simulink model "Copy_of_Q7Speed_Controller"  (R2013a)
settings: Solver=ode45  StartTime=0.0  StopTime=0.5  MaxStep=1e-4  RelTol=1e-3
values from neighbouring files (symbols this model uses):
  Km = (P/2)*(Kt/Bt)    (= 37.1743988584)    [Q1.m]    (also in Q4.m; Q5.m; Q6.m; Q8.m)
  La = Ls-(Lm*Lm/Lr)    (= 0.00366889047449)    [Q1.m]    (also in Q4.m; Q5.m; Q6.m; Q8.m)
  Ls = 0.0553    [Q1.m]    (also in Q4.m; Q5.m; Q6.m; Q8.m)
  Ra = Rs+Rr*(Ls/Lr)    (= 0.457519086693)    [Q1.m]    (also in Q4.m; Q5.m; Q6.m; Q8.m)
  Tm = J/Bt    (= 0.33)    [Q1.m]    (also in Q4.m; Q5.m; Q6.m; Q8.m)
undefined symbols (not defined in the file or in its folder): ids
settings Model: Creator=Sony  LastModifiedBy=Sony

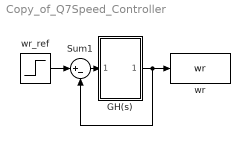
== system Copy_of_Q7Speed_Controller ==
  GH(s) : Subsystem
  Sum1 : Sum  Inputs=|+-
  wr : ToWorkspace  VariableName=wr  SampleTime=-1  SaveFormat=Timeseries
  wr_ref : Step  Time=0  After=1*0.05  SampleTime=0
  wires:
  wr_ref/1 -> Sum1/1
  Sum1/1 -> GH(s)/1(In1)
  GH(s)/1(Out1) -> Sum1/2, wr/1

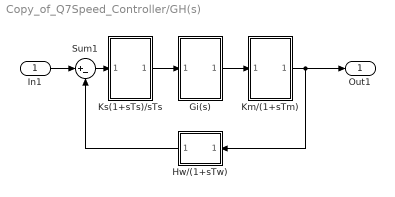
== system Copy_of_Q7Speed_Controller/GH(s) ==
  In1 : Inport
  Gi(s) : Subsystem
  Hw/(1+sTw) : Subsystem
  Km/(1+sTm) : Subsystem
  Ks(1+sTs)/sTs : Subsystem
  Sum1 : Sum  Inputs=|+-
  Out1 : Outport
  wires:
  In1/1 -> Sum1/1
  Km/(1+sTm)/1(Out1) -> Out1/1, Hw/(1+sTw)/1(In1)
  Ks(1+sTs)/sTs/1(Out1) -> Gi(s)/1(In1)
  Gi(s)/1(Out1) -> Km/(1+sTm)/1(In1)
  Hw/(1+sTw)/1(Out1) -> Sum1/2
  Sum1/1 -> Ks(1+sTs)/sTs/1(In1)

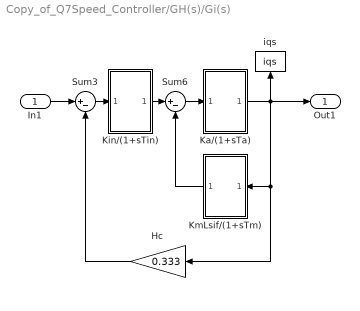
== system Copy_of_Q7Speed_Controller/GH(s)/Gi(s) ==
  In1 : Inport
  Hc : Gain  Gain=0.333
  Ka/(1+sTa) : Subsystem
  Kin/(1+sTin) : Subsystem
  KmLsif/(1+sTm) : Subsystem
  Sum3 : Sum  Inputs=|+-
  Sum6 : Sum  Inputs=|+-
  iqs : ToWorkspace  VariableName=iqs  SampleTime=-1  SaveFormat=Timeseries
  Out1 : Outport
  wires:
  Hc/1 -> Sum3/2
  In1/1 -> Sum3/1
  Sum6/1 -> Ka/(1+sTa)/1(In1)
  KmLsif/(1+sTm)/1(Out1) -> Sum6/2
  Ka/(1+sTa)/1(Out1) -> Out1/1, KmLsif/(1+sTm)/1(In1), Hc/1, iqs/1
  Sum3/1 -> Kin/(1+sTin)/1(In1)
  Kin/(1+sTin)/1(Out1) -> Sum6/1

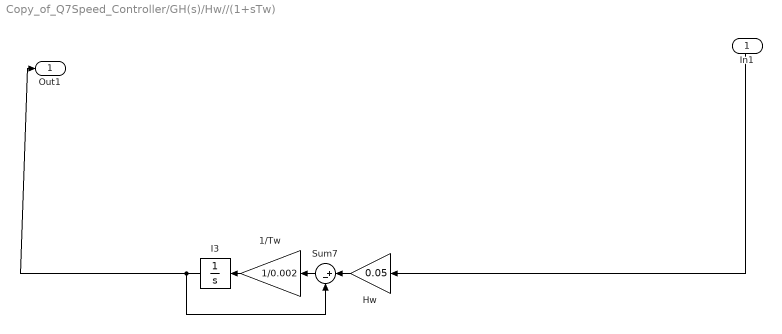
== system Copy_of_Q7Speed_Controller/GH(s)/Hw//(1+sTw) ==
  In1 : Inport
  1/Tw : Gain  Gain=1/0.002
  Hw : Gain  Gain=0.05
  I3 : Integrator
  Sum7 : Sum  Inputs=|+-
  Out1 : Outport
  wires:
  Hw/1 -> Sum7/1
  I3/1 -> Out1/1, Sum7/2
  1/Tw/1 -> I3/1
  Sum7/1 -> 1/Tw/1
  In1/1 -> Hw/1

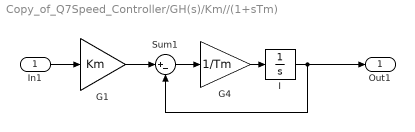
== system Copy_of_Q7Speed_Controller/GH(s)/Km//(1+sTm) ==
  In1 : Inport
  G1 : Gain  Gain=Km
  G4 : Gain  Gain=1/Tm
  I : Integrator
  Sum1 : Sum  Inputs=|+-
  Out1 : Outport
  wires:
  G4/1 -> I/1
  G1/1 -> Sum1/1
  Sum1/1 -> G4/1
  I/1 -> Out1/1, Sum1/2
  In1/1 -> G1/1

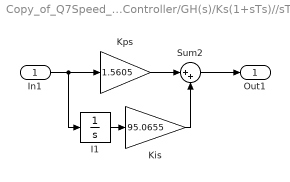
== system Copy_of_Q7Speed_Controller/GH(s)/Ks(1+sTs)//sTs ==
  In1 : Inport
  I1 : Integrator
  Kis : Gain  Gain=95.0655
  Kps : Gain  Gain=1.5605
  Sum2 : Sum  Inputs=|++
  Out1 : Outport
  wires:
  In1/1 -> I1/1, Kps/1
  I1/1 -> Kis/1
  Kps/1 -> Sum2/1
  Kis/1 -> Sum2/2
  Sum2/1 -> Out1/1

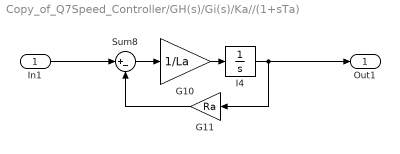
== system Copy_of_Q7Speed_Controller/GH(s)/Gi(s)/Ka//(1+sTa) ==
  In1 : Inport
  G10 : Gain  Gain=1/La
  G11 : Gain  Gain=Ra
  I4 : Integrator
  Sum8 : Sum  Inputs=|+-
  Out1 : Outport
  wires:
  G11/1 -> Sum8/2
  I4/1 -> Out1/1, G11/1
  Sum8/1 -> G10/1
  G10/1 -> I4/1
  In1/1 -> Sum8/1

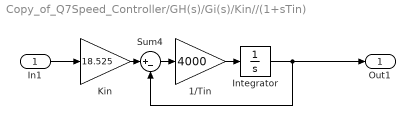
== system Copy_of_Q7Speed_Controller/GH(s)/Gi(s)/Kin//(1+sTin) ==
  In1 : Inport
  1/Tin : Gain  Gain=4000
  Integrator : Integrator
  Kin : Gain  Gain=18.525
  Sum4 : Sum  Inputs=|+-
  Out1 : Outport
  wires:
  Sum4/1 -> 1/Tin/1
  Kin/1 -> Sum4/1
  1/Tin/1 -> Integrator/1
  In1/1 -> Kin/1
  Integrator/1 -> Out1/1, Sum4/2

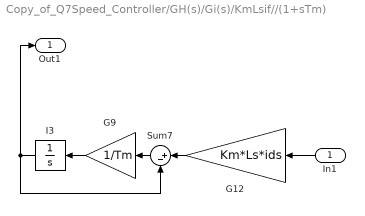
== system Copy_of_Q7Speed_Controller/GH(s)/Gi(s)/KmLsif//(1+sTm) ==
  In1 : Inport
  G12 : Gain  Gain=Km*Ls*ids
  G9 : Gain  Gain=1/Tm
  I3 : Integrator
  Sum7 : Sum  Inputs=|+-
  Out1 : Outport
  wires:
  Sum7/1 -> G9/1
  I3/1 -> Out1/1, Sum7/2
  G12/1 -> Sum7/1
  G9/1 -> I3/1
  In1/1 -> G12/1
